simulink model "CompleteModel"  (R2015a)
settings: Solver=ode23  StartTime=0.0  StopTime=20000  RelTol=1e-3
StopFcn:
  | stopfun
undefined symbols (not defined in the file or in its folder): Settings
libraries: Battery_Unipi x6, simulink x2
settings Model: TunableVars=Bp2,Bp3,Cl,Cs,N,Nbits,OCV_LUT,Qr,R0,Rl,Rs,T,dec_fact,ocv,params_bp,sampletime,soc_bp,soc_init  TunableVarsStorageClass=Auto,Auto,Auto,Auto,Auto,Auto,Auto,Auto,Auto,Auto,Auto,Auto,Auto,Auto,Auto,Auto,Auto,Auto  TunableVarsTypeQualifier=,,,,,,,,,,,,,,,,,  Creator=Rocco  LastModifiedBy=pc2
settings OptimizationCC: InlineParams=on  SimCompilerOptimization=on
settings DebuggingCC: ReadBeforeWriteMsg=DisableAll  WriteAfterWriteMsg=DisableAll  WriteAfterReadMsg=DisableAll  MultiTaskDSMMsg=none
settings ModelReferenceCC: UpdateModelReferenceTargets=IfOutOfDate
settings SFSimCC: SFSimEcho=off

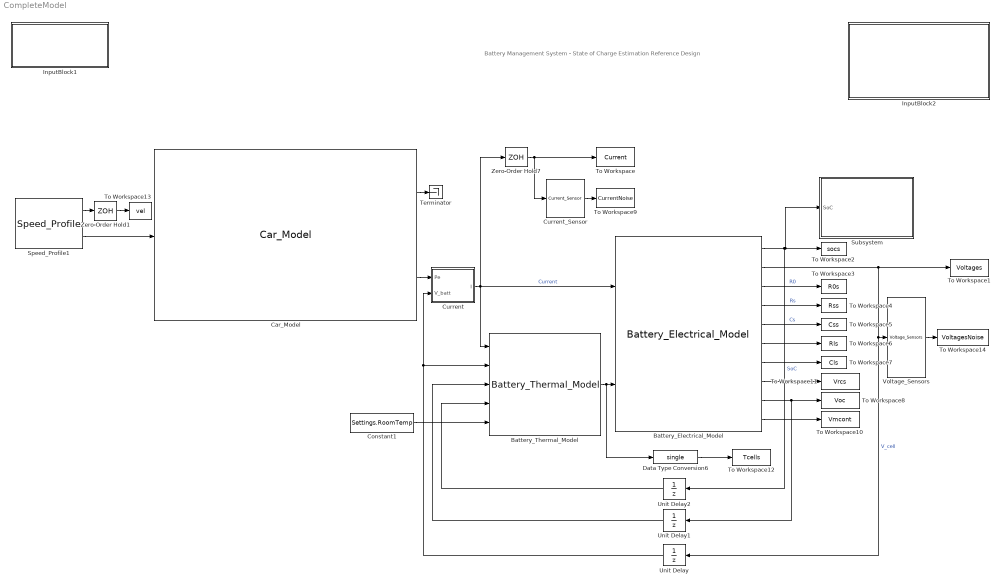
== system CompleteModel ==
  note: Battery Management System - State of Charge Estimation Reference Design
  Battery_Electrical_Model : Battery_Unipi/Battery_Electrical_Model  N=Settings.N  sampletime=Settings.sampletime  Qbattery=Settings.Q  ocv=Settings.ocv  soc_bp=Settings.soc_bp  params_bp=Settings.params_bp  Ro=Settings.R0lut3d  Rs=Settings.Rslut3d  Cs=Settings.Cslut3d  Rl=Settings.Rllut3d  Cl=Settings.Cllut3d  SoC0=Settings.SoCi  Bp2=Settings.Bp2  Bp3=Settings.Bp3
      link override Cell_Model_therm: R0=Ro
  Battery_Thermal_Model : Battery_Unipi/Battery_Thermal_Model  M=Settings.N/Settings.Strings  Rthca=Settings.ThermRthca  Rthcc=Settings.ThermRthcc  Cth=Settings.ThermCap  Ta=Settings.InitTemp  sampletime=Settings.sampletime
  Car_Model : Battery_Unipi/Car_Model  M=1525  S=2.27  Cx=0.29  alphaR=0.01  roair=1.2  n_wheel=0.7  n_reg=0.5
  Constant1 : Constant  Value=Settings.RoomTemp
  Current : Subsystem
  Current_Sensor : Battery_Unipi/Current_Sensor  sampletime=Settings.sampletime  noisevariance=Settings.CurrVar  Nbits=Settings.CurrNbits  FS=Settings.CurrFS  Offset=Settings.CurrOff
  Data Type Conversion6 : DataTypeConversion  OutDataTypeStr=single
  InputBlock1 : Subsystem
      mask DialogControl altera Prompt: www.altera.com
      mask Display: image('altera-logo-v3.png')
  InputBlock2 : Subsystem
      mask DialogControl altera Prompt: www.unipi.it
      mask Display: image('unipi.jpg')
  Speed_Profile1 : Battery_Unipi/Speed_Profile  selector=Settings.profile
  Subsystem : Subsystem
      mask Display:
      | image('stop.png')
      | port_label('input', 1, 'SoC')
  Terminator : Terminator
  To Workspace : ToWorkspace  VariableName=Current  SaveFormat=Timeseries  SampleTime=-1
  To Workspace1 : ToWorkspace  VariableName=Voltages  SaveFormat=Timeseries  SampleTime=-1
  To Workspace10 : ToWorkspace  VariableName=Vmcont  SaveFormat=Timeseries  SampleTime=-1
      settings: Decimation=10
  To Workspace11 : ToWorkspace  VariableName=Vrcs  SaveFormat=Timeseries  SampleTime=-1
      settings: Decimation=10
  To Workspace12 : ToWorkspace  VariableName=Tcells  SaveFormat=Timeseries  SampleTime=-1
      settings: Decimation=10
  To Workspace13 : ToWorkspace  VariableName=vel  SaveFormat=Timeseries  SampleTime=-1
  To Workspace14 : ToWorkspace  VariableName=VoltagesNoise  SaveFormat=Timeseries  SampleTime=-1
  To Workspace2 : ToWorkspace  VariableName=socs  SaveFormat=Timeseries  SampleTime=-1
  To Workspace3 : ToWorkspace  VariableName=R0s  SaveFormat=Timeseries  SampleTime=-1
      settings: Decimation=10
  To Workspace4 : ToWorkspace  VariableName=Rss  SaveFormat=Timeseries  SampleTime=-1
      settings: Decimation=10
  To Workspace5 : ToWorkspace  VariableName=Css  SaveFormat=Timeseries  SampleTime=-1
      settings: Decimation=10
  To Workspace6 : ToWorkspace  VariableName=Rls  SaveFormat=Timeseries  SampleTime=-1
      settings: Decimation=10
  To Workspace7 : ToWorkspace  VariableName=Cls  SaveFormat=Timeseries  SampleTime=-1
      settings: Decimation=10
  To Workspace8 : ToWorkspace  VariableName=Voc  SaveFormat=Timeseries  SampleTime=-1
      settings: Decimation=10
  To Workspace9 : ToWorkspace  VariableName=CurrentNoise  SaveFormat=Timeseries  SampleTime=-1
  Unit Delay : UnitDelay  InitialCondition=4.16  SampleTime=Settings.sampletime
  Unit Delay1 : UnitDelay  InitialCondition=4.16  SampleTime=Settings.sampletime
  Unit Delay2 : UnitDelay  InitialCondition=Settings.SoCi(1)  SampleTime=Settings.sampletime
  Voltage_Sensors : Battery_Unipi/Voltage_Sensors  sampletime=Settings.sampletime  noisevariance=Settings.VoltVar  Nbits=Settings.VoltNbits  FS=Settings.VoltFS  Offset=Settings.VoltOff
  Zero-Order Hold1 : ZeroOrderHold  SampleTime=Settings.sampletime
  Zero-Order Hold7 : ZeroOrderHold  SampleTime=Settings.sampletime
  wires:
  Car_Model/1 -> Terminator/1
  Battery_Electrical_Model/1 -> Unit Delay2/1, Subsystem/1(SoC), To Workspace2/1  "SoC"
  Battery_Electrical_Model/2 -> To Workspace1/1, Voltage_Sensors/1, Unit Delay/1  "V_cell"
  Battery_Electrical_Model/5 -> To Workspace5/1  "Cs"
  Battery_Electrical_Model/3 -> To Workspace3/1  "R0"
  Battery_Electrical_Model/4 -> To Workspace4/1  "Rs"
  Battery_Electrical_Model/8 -> To Workspace11/1
  Data Type Conversion6/1 -> To Workspace12/1
  Battery_Electrical_Model/6 -> To Workspace6/1
  Battery_Electrical_Model/7 -> To Workspace7/1
  Car_Model/2 -> Current/1(Pe)
  Zero-Order Hold1/1 -> To Workspace13/1
  Speed_Profile1/1 -> Zero-Order Hold1/1
  Speed_Profile1/2 -> Car_Model/1
  Zero-Order Hold7/1 -> To Workspace/1, Current_Sensor/1
  Current_Sensor/1 -> To Workspace9/1
  Current/1(I) -> Battery_Electrical_Model/1, Battery_Thermal_Model/1, Zero-Order Hold7/1  "Current"
  Battery_Electrical_Model/10 -> To Workspace10/1
  Battery_Electrical_Model/9 -> Unit Delay1/1, To Workspace8/1
  Voltage_Sensors/1 -> To Workspace14/1
  Battery_Thermal_Model/1 -> Battery_Electrical_Model/2, Data Type Conversion6/1
  Constant1/1 -> Battery_Thermal_Model/5
  Unit Delay/1 -> Battery_Thermal_Model/2, Current/2(V_batt)
  Unit Delay1/1 -> Battery_Thermal_Model/3
  Unit Delay2/1 -> Battery_Thermal_Model/4

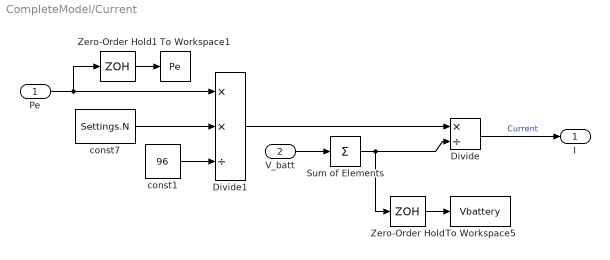
== system CompleteModel/Current ==
  Pe : Inport
  V_batt : Inport  Port=2
  Divide : Product  Inputs=*/
  Divide1 : Product  Inputs=**/
  Sum of Elements : Sum  Inputs=+
  To Workspace1 : ToWorkspace  VariableName=Pe  SaveFormat=Timeseries  SampleTime=-1
      settings: Decimation=10
  To Workspace5 : ToWorkspace  VariableName=Vbattery  SaveFormat=Timeseries  SampleTime=-1
      settings: Decimation=10
  Zero-Order Hold : ZeroOrderHold  SampleTime=Settings.sampletime
  Zero-Order Hold1 : ZeroOrderHold  SampleTime=Settings.sampletime
  const1 : Constant  Value=96  OutDataTypeStr=single  SampleTime=Inf
  const7 : Constant  Value=Settings.N  OutDataTypeStr=single  SampleTime=Inf
  I : Outport
  wires:
  Divide1/1 -> Divide/1
  const1/1 -> Divide1/3
  V_batt/1 -> Sum of Elements/1
  Sum of Elements/1 -> Divide/2, Zero-Order Hold/1
  const7/1 -> Divide1/2
  Pe/1 -> Zero-Order Hold1/1, Divide1/1
  Divide/1 -> I/1  "Current"
  Zero-Order Hold/1 -> To Workspace5/1
  Zero-Order Hold1/1 -> To Workspace1/1

== system CompleteModel/InputBlock1 ==

== system CompleteModel/InputBlock2 ==

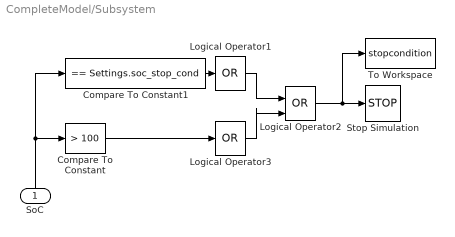
== system CompleteModel/Subsystem ==
  SoC : Inport
  Compare To Constant : simulink/Logic and Bit Operations/Compare To Constant  relop=>  const=100  OutDataTypeStr=boolean
  Compare To Constant1 : simulink/Logic and Bit Operations/Compare To Constant  relop===  const=Settings.soc_stop_cond  OutDataTypeStr=boolean  ZeroCross=off
  Logical Operator1 : Logic  Operator=OR  Inputs=1  IconShape=distinctive  AllPortsSameDT=off  OutDataTypeStr=boolean
  Logical Operator2 : Logic  Operator=OR  IconShape=distinctive  AllPortsSameDT=off  OutDataTypeStr=boolean
  Logical Operator3 : Logic  Operator=OR  Inputs=1  IconShape=distinctive  AllPortsSameDT=off  OutDataTypeStr=boolean
  Stop Simulation : Stop
  To Workspace : ToWorkspace  VariableName=stopcondition  SaveFormat=Timeseries  SampleTime=-1
  wires:
  Compare To Constant/1 -> Logical Operator3/1
  Compare To Constant1/1 -> Logical Operator1/1
  SoC/1 -> Compare To Constant/1, Compare To Constant1/1
  Logical Operator2/1 -> To Workspace/1, Stop Simulation/1
  Logical Operator3/1 -> Logical Operator2/2
  Logical Operator1/1 -> Logical Operator2/1
